simulink model "feedback_control_digital"  (R2015a)
settings: Solver=ode45  StartTime=0.0  StopTime=t_stop  MaxStep=1e-5  MinStep=1e-6  RelTol=1e-3
values from neighbouring files (symbols this model uses):
  delta_a = 0    [automatic_control_lab6_exercise4.m]
  delta_t = 0    [automatic_control_lab6_exercise4.m]
  delta_y = 0    [automatic_control_lab6_exercise4.m]
  rho = 2    [automatic_control_lab6_exercise4.m]
  Ts = 0.02    [automatic_control_lab6_exercise4.m]
  w_t = 90    [automatic_control_lab6_exercise4.m]
  w_y = 0    [automatic_control_lab6_exercise4.m]
libraries: cstblocks x2
settings Model: Creator=Berk Delibalta  LastModifiedBy=Berk Delibalta
settings SolverCC: InitialStep=1e-6

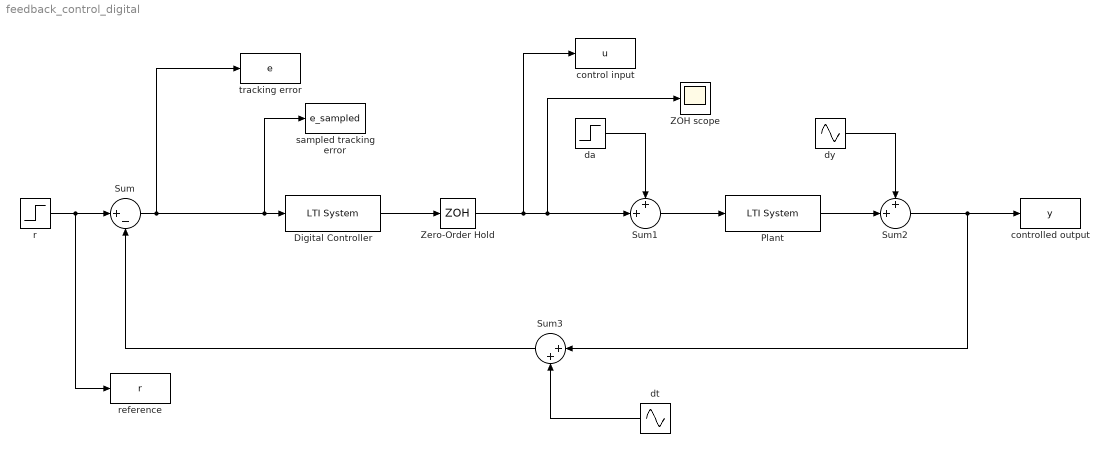
== system feedback_control_digital ==
  Digital Controller : cstblocks/LTI System  sys=Cd  IC=[]
  "Plant " : cstblocks/LTI System  sys=G  IC=[]
  Sum : Sum  Inputs=|+-
  Sum1 : Sum  Inputs=++|
  Sum2 : Sum  Inputs=++|
  Sum3 : Sum  Inputs=|++
  "ZOH scope " : Scope
  Zero-Order Hold : ZeroOrderHold  SampleTime=Ts
  "control input " : ToWorkspace  VariableName=u  SaveFormat=Timeseries  SampleTime=-1
  "controlled output " : ToWorkspace  VariableName=y  SaveFormat=Timeseries  SampleTime=-1
  da : Step  Time=0  After=delta_a  SampleTime=0
  dt : Sin  Amplitude=delta_t  Frequency=w_t  SampleTime=0
  dy : Sin  Amplitude=delta_y  Bias=delta_y  Frequency=w_y  SampleTime=0
  r : Step  Time=0  After=rho  SampleTime=0
  "reference " : ToWorkspace  VariableName=r  SaveFormat=Timeseries  SampleTime=-1
  "sampled tracking error " : ToWorkspace  VariableName=e_sampled  SaveFormat=Timeseries  SampleTime=-1
  "tracking error " : ToWorkspace  VariableName=e  SaveFormat=Timeseries  SampleTime=-1
  wires:
  Sum/1 -> "tracking error "/1, "sampled tracking error "/1, Digital Controller/1
  Digital Controller/1 -> Zero-Order Hold/1
  Zero-Order Hold/1 -> Sum1/2, "ZOH scope "/1, "control input "/1
  da/1 -> Sum1/1
  Sum1/1 -> "Plant "/1
  "Plant "/1 -> Sum2/2
  dy/1 -> Sum2/1
  Sum2/1 -> Sum3/1, "controlled output "/1
  Sum3/1 -> Sum/2
  dt/1 -> Sum3/2
  r/1 -> "reference "/1, Sum/1
